simulink model "Simulation_model_islanded"  (R2021a)
settings: Solver=ode23t  StartTime=0.0  StopTime=6  FixedStep=T  RelTol=1e-3
values from neighbouring files (symbols this model uses):
  C_dc = Cb*c_dc_pu    [parameters.m]
  C_f = Cb*c_f_pu    [parameters.m]
  f_SM = fb    (= 50)    [parameters.m]
  fb = 50    [parameters.m]
  ff_SM = 0.01322    [parameters.m]
  Ib = 2/3*Sb/Vb    [parameters.m]
  Ib_dc = Sb/Vb_dc    [parameters.m]
  ic_SM = 0.8    [parameters.m]
  K_ad = 1.5    [parameters.m]
  K_ffv = 0    [parameters.m]
  K_ic = K_pc/T_1    [parameters.m]
  K_idc = K_pdc/T_idc    (= 250)    [parameters.m]
  K_iPLL = a^2*T_fPLL    (= 0.09)    [parameters.m]
  K_iv = K_pv/T_iv    (= 92.0050761421)    [parameters.m]
  K_iv_SM = K_pv_SM/T_iv_SM    (= 70)    [parameters.m]
  K_omega = 20    [parameters.m]
  K_omega_SM = 40    [parameters.m]
  K_pc = l_f_pu/(4*pi*fb*T_sum)    (= 1.27323954474)    [parameters.m]
  K_pdc = 25    [parameters.m]
  K_pPLL = 1/(a*2*pi*T_fPLL)    (= 5.30516476973)    [parameters.m]
  K_pv = 0.29    [parameters.m]
  K_pv_SM = 35    [parameters.m]
  K_vco = 2*pi    (= 6.28318530718)    [parameters.m]
  Kd = 40    [parameters.m]
  Kq = 0.1    [parameters.m]
  Kq_SM = 0.1    [parameters.m]
  L_f = Lb*l_f_pu    [parameters.m]
  l_f_pu = 0.08    [parameters.m]
  lf1f = 0    [parameters.m]
  lfd_SM = 0.531    [parameters.m]
  llkd = 2.655    [parameters.m]
  llkq1 = 0.2408    [parameters.m]
  lls_SM = 0.08    [parameters.m]
  lmd_SM = 2.81    [parameters.m]
  lmq_SM = 1.64    [parameters.m]
  omega_ad = 50    [parameters.m]
  omega_b = 2*pi*fb    (= 314.159265359)    [parameters.m]
  omega_d = 5    [parameters.m]
  omega_qf = 200    [parameters.m]
  omega_qf_SM = 200    [parameters.m]
  omega_vf = 200    [parameters.m]
  p_h = 0.1    [parameters.m]
  pp_SM = 2    [parameters.m]
  R_lf = Rb*r_lf_pu    [parameters.m]
  rfd_SM = 0.004319    [parameters.m]
  rkd = 0.2343    [parameters.m]
  rkq1 = 0.03365    [parameters.m]
  rs_SM = 0.01524    [parameters.m]
  S_SM = Sb    (= 1000000)    [parameters.m]
  Sb = 1e6    (= 1000000)    [parameters.m]
  T = 1e-4    (= 0.0001)    [parameters.m]
  T_fPLL = 10e-3    (= 0.01)    [parameters.m]
  T_gt_SM = 0.5    [parameters.m]
  Ta = 4    [parameters.m]
  v_dc_ref = 1    [parameters.m]
  V_SM = V    (= 690)    [parameters.m]
  Vb = V*sqrt(2)/sqrt(3)    [parameters.m]
  Vb_dc = Vb*2    [parameters.m]
undefined symbols (not defined in the file or in its folder): D11, Delta
libraries: simulink_extras x18, spsDiodeLib x12, spsThreePhaseVIMeasurementLib x9, spsThreePhaseSeriesRLCBranchLib x7, spsPower3phInstantaneousLib x5, spsVoltageMeasurementLib x3, spsControlledCurrentSourceLib x2, spsThreePhaseParallelRLCLoadLib x2, spsThreePhaseBreakerLib x2, spsUniversalBridgeLib x2, spsDCVoltageSourceLib x1, spsGroundLib x1
(part 1 of 2)
settings Model: Creator=HLunn  LastModifiedBy=HLunn

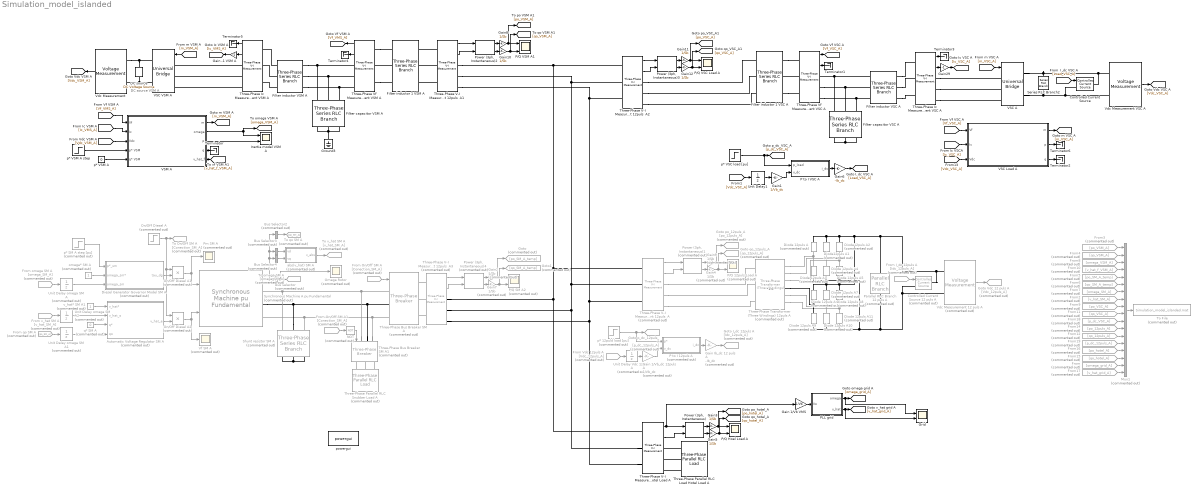
== system Simulation_model_islanded ==
  note: *1.6
  note: DC source
      | VSM A
  Automatic Voltage Regulator SM A : Subsystem  Commented=on
  Bus Selector : BusSelector  Commented=on  OutputSignals="Mechanical.Rotor speed  wm (pu)"  OutputAsBus=on
  Bus Selector2 : BusSelector  Commented=on  OutputSignals="Output reactive power  Qeo (pu)"  OutputAsBus=on
  Bus Selector3 : BusSelector  Commented=on  OutputSignals="dq0 components.Stator voltage  vd (pu)"  OutputAsBus=on
  Bus Selector4 : BusSelector  Commented=on  OutputSignals="dq0 components.Stator voltage  vq (pu)"  OutputAsBus=on
  Controlled Current Source : spsControlledCurrentSourceLib/Controlled Current Source  Initialize=on  Source_Type=DC  Amplitude=0  Phase=0  Frequency=0  Measurements=None
  Controlled Current Source 12 puls A : spsControlledCurrentSourceLib/Controlled Current Source  Commented=on  Initialize=on  Source_Type=DC  Amplitude=0  Phase=0  Frequency=0  Measurements=None
  DC source : spsDCVoltageSourceLib/DC Voltage Source  Amplitude=Vb_dc  Measurements=None
  Diesel Generator Governor Model SM A : Subsystem  Commented=on
  Diode 12puls A{,3..11} (10 alike) : spsDiodeLib/Diode  Commented=on  Ron=0.001  Lon=0  Vf=0.8  IC=0  UseSnubber=0  Rs=500  Cs=250e-9  Measurements=off
  Diode12puls A1 : spsDiodeLib/Diode  Commented=on  Ron=0.001  Lon=0  Vf=0.8  IC=0  UseSnubber=0  Rs=500  Cs=250e-9  Measurements=off
  Diode12puls A2 : spsDiodeLib/Diode  Commented=on  Ron=0.001  Lon=0  Vf=0.8  IC=0  UseSnubber=0  Rs=500  Cs=250e-9  Measurements=off
  Filter capacitor VSC A : spsThreePhaseSeriesRLCBranchLib/Three-Phase Series RLC Branch  LConnTagsString=A|B|C  RConnTagsString=A|B|C  BranchType=RC  Resistance=R_lf  Inductance=L_f  Capacitance=C_f  Measurements=None
  Filter capacitor VSM A : spsThreePhaseSeriesRLCBranchLib/Three-Phase Series RLC Branch  LConnTagsString=A|B|C  RConnTagsString=A|B|C  BranchType=RC  Resistance=R_lf  Inductance=L_f  Capacitance=C_f  Measurements=None
  Filter inductor VSC A : spsThreePhaseSeriesRLCBranchLib/Three-Phase Series RLC Branch  LConnTagsString=A|B|C  RConnTagsString=A|B|C  BranchType=RL  Resistance=R_lf  Inductance=L_f  Capacitance=1e-6  Measurements=None
  Filter inductor VSM A : spsThreePhaseSeriesRLCBranchLib/Three-Phase Series RLC Branch  LConnTagsString=A|B|C  RConnTagsString=A|B|C  BranchType=RL  Resistance=R_lf  Inductance=L_f  Capacitance=1e-6  Measurements=None
  Filter inductor 1 VSC A : spsThreePhaseSeriesRLCBranchLib/Three-Phase Series RLC Branch  LConnTagsString=A|B|C  RConnTagsString=A|B|C  BranchType=RL  Resistance=R_lf  Inductance=L_f  Capacitance=1e-6  Measurements=None
  Filter inductor 1 VSM A : spsThreePhaseSeriesRLCBranchLib/Three-Phase Series RLC Branch  LConnTagsString=A|B|C  RConnTagsString=A|B|C  BranchType=RL  Resistance=R_lf  Inductance=L_f  Capacitance=1e-6  Measurements=None
  From : From  Commented=on  GotoTag=omega_grid_A
  From I_dc 12puls A : From  Commented=on  GotoTag=Idc_12puls_A
  From On/Off SM A : From  Commented=on  GotoTag=Conection_SM_A
  From On/Off SM A1 : From  Commented=on  GotoTag=Conection_SM_A
  From Vdc 12puls A : From  Commented=on  GotoTag=Vdc_12puls_A
  From omega SM A : From  Commented=on  GotoTag=omega_SM_A
  From qo SM A : From  Commented=on  GotoTag=qo_SM_A
  From v_hat SM A : From  Commented=on  GotoTag=v_hat_SM_A
  From10 : From  Commented=on  GotoTag=v_hat_f_VSM_A
  From11 : From  Commented=on  GotoTag=qo_VSC_A
  From12 : From  Commented=on  GotoTag=qo_12puls_A
  From14 : From  Commented=on  GotoTag=po_12puls_A
  From15 : From  Commented=on  GotoTag=qo_hotel_A
  From16 : From  Commented=on  GotoTag=po_hotel_A
  From17 : From  Commented=on  GotoTag=v_hat_grid_A
  From18 : From  Commented=on  GotoTag=p_dc_VSC_A
  From19 : From  Commented=on  GotoTag=p_dc_12puls_A
  From2 : From  Commented=on  GotoTag=v_hat_SM_A
  From3 : From  Commented=on  GotoTag=po_VSM_A
  From4 : From  Commented=on  GotoTag=qo_VSM_A
  From5 : From  Commented=on  GotoTag=po_SM_A_temp
  From6 : From  Commented=on  GotoTag=qo_SM_A_temp
  From7 : From  Commented=on  GotoTag=omega_SM_A
  From8 : From  Commented=on  GotoTag=omega_VSM_A
  From9 : From  Commented=on  GotoTag=po_VSC_A
  Gain -1 VSM A : Gain  Gain=-1
  Gain 1/Vb VMS : Gain  Gain=1/Vb
  Gain 1/Vb_dc 12puls A : Gain  Commented=on  Gain=1/Vb_dc
  Gain Ib_dc 12 puls A : Gain  Commented=on  Gain=-Ib_dc
  Gain1 : Gain  Gain=1/Vb_dc
  Gain{3,5,8,10..12} (6 alike) : Gain  Gain=1/Sb
  Gain{2,4,7,9} (4 alike) : Gain  Commented=on  Gain=1/Sb
  Gain29 : Gain  Gain=-1
  Gain6 : Gain  Gain=-Ib_dc
  Goto : Goto  Commented=on  GotoTag=po_SM_A_temp
  Goto I_dc 12puls A : Goto  Commented=on  GotoTag=Idc_12puls_A
  Goto Vdc 12 puls A : Goto  Commented=on  GotoTag=Vdc_12puls_A
  Goto p_dc_12puls_A : Goto  Commented=on  GotoTag=p_dc_12puls_A
  Goto po_12puls_A : Goto  Commented=on  GotoTag=po_12puls_A
  Goto qo_12puls_A : Goto  Commented=on  GotoTag=qo_12puls_A
  Goto1 : Goto  Commented=on  GotoTag=qo_SM_A_temp
  Grid : Scope  NumInputPorts=2
  Ground3 : spsGroundLib/Ground  LConnTagsString=a
  Inertia model VSM A : Scope  NumInputPorts=2
  Mux1 : Mux  Commented=on  Inputs=18
  NOT : Logic  Commented=on  Operator=NOT  IconShape=distinctive  AllPortsSameDT=off  OutDataTypeStr=boolean
  Omega Rotor : Scope  Commented=on
  On/Off Diesel A : Step  Commented=on  Time=4.002  Before=1  After=0  SampleTime=0
  On/Off Diesel A1 : Product  Commented=on  Inputs=**
  On/Off Diesel A2 : Product  Commented=on  Inputs=**
  P to I VSC A : Subsystem
  P to I 12puls A : Subsystem  Commented=on
  P/Q 12puls Load A : Scope  Commented=on  NumInputPorts=2
  P/Q Hoel Load A : Scope  NumInputPorts=2
  P/Q SM A2 : Scope  Commented=on  NumInputPorts=2
  P/Q VSC Load A : Scope  NumInputPorts=2
  P/Q VSM A1 : Scope  NumInputPorts=2
  PLL grid : Subsystem
  Parallel RLC Branch 12 puls A : spsParallelRLCBranchLib/Parallel RLC Branch  Commented=on  LConnTagsString=a  RConnTagsString=__new0  BranchType=C  Resistance=1e3  Inductance=1e-3  SetiL0=off  InitialCurrent=0  Capacitance=C_dc  Setx0=on  InitialVoltage=Vb_dc  Measurements=None
  Pm SM A : Scope  Commented=on
  "Power (3ph, Instantaneous)" : spsPower3phInstantaneousLib/Power (3ph, Instantaneous)
  "Power (3ph, Instantaneous)1" : spsPower3phInstantaneousLib/Power (3ph, Instantaneous)  Commented=on
  "Power (3ph, Instantaneous)2" : spsPower3phInstantaneousLib/Power (3ph, Instantaneous)
  "Power (3ph, Instantaneous)3" : spsPower3phInstantaneousLib/Power (3ph, Instantaneous)
  "Power (3ph, Instantaneous)4" : spsPower3phInstantaneousLib/Power (3ph, Instantaneous)  Commented=on
  Series RLC Branch2 : spsSeriesRLCBranchLib/Series RLC Branch  LConnTagsString=__new0  RConnTagsString=__new0  BranchType=C  Resistance=0  Inductance=0  SetiL0=off  InitialCurrent=0  Capacitance=C_dc  Setx0=on  InitialVoltage=Vb_dc  Measurements=None
  Shunt resistor SM A : spsThreePhaseSeriesRLCBranchLib/Three-Phase Series RLC Branch  Commented=on  LConnTagsString=A|B|C  RConnTagsString=A|B|C  BranchType=R  Resistance=1e6  Inductance=L_f  Capacitance=C_f  Measurements=None
  Synchronous Machine A pu Fundamental : spsSynchronousMachinepuFundamentalLib/Synchronous Machine pu Fundamental  Commented=on  PresetModel=No  MechanicalLoad=Mechanical power Pm  ShowDetailedParameters=on  RotorType=Salient-pole  Units=per unit fundamental parameters  MeasurementBus=off  NominalParameters=[S_SM V_SM f_SM]  Stator=[rs_SM lls_SM lmd_SM lmq_SM lf1f]  Field=[rfd_SM lfd_SM]  Dampers2=[0.0652, 0.5134, 0.0287, 0.2553, 7.765e-3, 0.9167 ]  Dampers1=[rkd llkd rkq1 llkq1]  Mechanical=[ic_SM ff_SM pp_SM]  PolePairs=20  InitialConditions="[ 0  0  0  0  0  0  0  0  1 ]"  SetSaturation=off  Saturation=[0.6404,0.7127,0.8441,0.9214,0.9956,1.082,1.19,1.316,1.457;0.7,0.7698,0.8872,0.9466,0.9969,1.046,1.1,1.151,1.201]  LoadFlowParameters=[1,0,0,0,0]  TsPowergui=0  TsBlock=-1  IterativeModel=Trapezoidal non iterative  IterativeDiscreteModel=Trapezoidal non iterative  BusType=PV  Pref=0  Qref=0  Qmin=-inf  Qmax=inf  PLF=0  QLF=0
      settings: SourceProductBaseCode=PS
  Terminator{,1..6} (7 alike) : Terminator
  Three-Phase Ic Measurement VSC A : spsThreePhaseVIMeasurementLib/Three-Phase V-I Measurement  VoltageMeasurement=phase-to-ground  SetLabelV=off  LabelV=V_cv  Vpu=off  VpuLL=off  CurrentMeasurement=yes  SetLabelI=off  LabelI=I_cv  Ipu=off  Pbase=Sb  Vbase=V  OutputType=Complex  PhasorSimulation=off  PSBequivalent=0
  Three-Phase Ic Measurement VSM A : spsThreePhaseVIMeasurementLib/Three-Phase V-I Measurement  VoltageMeasurement=phase-to-ground  SetLabelV=off  LabelV=V_cv  Vpu=off  VpuLL=off  CurrentMeasurement=yes  SetLabelI=off  LabelI=I_cv  Ipu=off  Pbase=Sb  Vbase=V  OutputType=Complex  PhasorSimulation=off  PSBequivalent=0
  Three-Phase Parallel RLC Snubber Load A : spsThreePhaseParallelRLCLoadLib/Three-Phase Parallel RLC Load  Commented=on  LConnTagsString=A|B|C  Configuration=Y (floating)  NominalVoltage=690  Vabc=[1e3 1e3 1e3]  Vabcp=[1e3 1e3 1e3]  NominalFrequency=50  UnbalancedPower=off  ActivePower=Sb*0.5  InductivePower=0  CapacitivePower=0  Pabc=[10e3 9e3 11e3]  QLabc=[100 90 110]  QCabc=[100 90 110]  Pabcp=[10e3 9e3 11e3]  QLabcp=[100 90 110]  QCabcp=[100 90 110]  Measurements=None  LoadType=constant Z
  Three-Phase Parallel RLC Load Hotel Load A : spsThreePhaseParallelRLCLoadLib/Three-Phase Parallel RLC Load  LConnTagsString=A|B|C  Configuration=Y (floating)  NominalVoltage=690  Vabc=[1e3 1e3 1e3]  Vabcp=[1e3 1e3 1e3]  NominalFrequency=fb  UnbalancedPower=off  ActivePower=Sb*p_h  InductivePower=0  CapacitivePower=0  Pabc=[10e3 9e3 11e3]  QLabc=[100 90 110]  QCabc=[100 90 110]  Pabcp=[10e3 9e3 11e3]  QLabcp=[100 90 110]  QCabcp=[100 90 110]  Measurements=None  LoadType=constant Z
  Three-Phase Transformer (Three Windings) 12puls A : spsThreePhaseTransformerThreeWindingsLib/Three-Phase Transformer (Three Windings)  Commented=on  Winding1Connection=Y  Winding2Connection=Y  Winding3Connection=Delta (D11)  CoreType=Three single-phase transformers  SetSaturation=off  Hysteresis=off  DataFile='hysteresis'  SetInitialFlux=off  Measurements=None  UNITS=pu  NominalPower=[Sb , fb]  Winding1=[690 0.005 0.04]  Winding2=[690 0.005 0.03]  Winding3=[690 0.005 0.03]  Rm=100  Lm=100  L0=0.5  Saturation=[0 0;2.2531e-06 1278.3;0.00093879 1619.1]  InitialFluxes=[0.8 -0.8 0.7]  BreakLoop=off  DiscreteSolver=Trapezoidal iterative  DataType=off  TransfoNumber=1
      settings: SourceProductBaseCode=PS
  Three-Phase V-I Measurement 12puls  A : spsThreePhaseVIMeasurementLib/Three-Phase V-I Measurement  Commented=on  VoltageMeasurement=phase-to-ground  SetLabelV=off  LabelV=Vabc  Vpu=off  VpuLL=off  CurrentMeasurement=yes  SetLabelI=off  LabelI=Iabc  Ipu=off  Pbase=100e6  Vbase=500e3  OutputType=Complex  PhasorSimulation=off  PSBequivalent=0
  Three-Phase V-I Measurement 12puls  A1 : spsThreePhaseVIMeasurementLib/Three-Phase V-I Measurement  VoltageMeasurement=phase-to-ground  SetLabelV=off  LabelV=Vabc  Vpu=off  VpuLL=off  CurrentMeasurement=yes  SetLabelI=off  LabelI=Iabc  Ipu=off  Pbase=100e6  Vbase=500e3  OutputType=Complex  PhasorSimulation=off  PSBequivalent=0
  Three-Phase V-I Measurement 12puls  A2 : spsThreePhaseVIMeasurementLib/Three-Phase V-I Measurement  VoltageMeasurement=phase-to-ground  SetLabelV=off  LabelV=Vabc  Vpu=off  VpuLL=off  CurrentMeasurement=yes  SetLabelI=off  LabelI=Iabc  Ipu=off  Pbase=100e6  Vbase=500e3  OutputType=Complex  PhasorSimulation=off  PSBequivalent=0
  Three-Phase V-I Measurement 12puls  A3 : spsThreePhaseVIMeasurementLib/Three-Phase V-I Measurement  Commented=on  VoltageMeasurement=phase-to-ground  SetLabelV=off  LabelV=Vabc  Vpu=off  VpuLL=off  CurrentMeasurement=yes  SetLabelI=off  LabelI=Iabc  Ipu=off  Pbase=100e6  Vbase=500e3  OutputType=Complex  PhasorSimulation=off  PSBequivalent=0
  Three-Phase V-I Measurement Hotel Load A : spsThreePhaseVIMeasurementLib/Three-Phase V-I Measurement  VoltageMeasurement=phase-to-ground  SetLabelV=off  LabelV=Vabc  Vpu=off  VpuLL=off  CurrentMeasurement=yes  SetLabelI=off  LabelI=Iabc  Ipu=off  Pbase=100e6  Vbase=500e3  OutputType=Complex  PhasorSimulation=off  PSBequivalent=0
  Three-Phase Vf Measurement VSC A : spsThreePhaseVIMeasurementLib/Three-Phase V-I Measurement  VoltageMeasurement=phase-to-ground  SetLabelV=off  LabelV=Vabc  Vpu=off  VpuLL=off  CurrentMeasurement=yes  SetLabelI=off  LabelI=Iabc  Ipu=off  Pbase=100e6  Vbase=500e3  OutputType=Complex  PhasorSimulation=off  PSBequivalent=0
  Three-Phase Vf Measurement VSM A : spsThreePhaseVIMeasurementLib/Three-Phase V-I Measurement  VoltageMeasurement=phase-to-ground  SetLabelV=off  LabelV=Vabc  Vpu=off  VpuLL=off  CurrentMeasurement=yes  SetLabelI=off  LabelI=Iabc  Ipu=off  Pbase=100e6  Vbase=500e3  OutputType=Complex  PhasorSimulation=off  PSBequivalent=0
  Three-Phase Bus Breaker SM A : spsThreePhaseBreakerLib/Three-Phase Breaker  Commented=on  InitialState=closed  SwitchA=on  SwitchB=on  SwitchC=on  SwitchTimes=[1]  External=on  BreakerResistance=0.01  SnubberResistance=1e6  SnubberCapacitance=inf  Measurements=None
  Three-Phase Bus Breaker SM A1 : spsThreePhaseBreakerLib/Three-Phase Breaker  Commented=on  InitialState=open  SwitchA=on  SwitchB=on  SwitchC=on  SwitchTimes=[1]  External=on  BreakerResistance=0.01  SnubberResistance=1e6  SnubberCapacitance=inf  Measurements=None
  To File : ToFile  Commented=on  Filename=Simulation_model_islanded.mat  MatrixName=Simulation_model_islanded
  To On/Off SM A : Goto  Commented=on  GotoTag=Conection_SM_A
  To omega SM A : Goto  Commented=on  GotoTag=omega_SM_A
  To qo SM A : Goto  Commented=on  GotoTag=qo_SM_A
  To v_hat SM A : Goto  Commented=on  GotoTag=v_hat_SM_A
  Unit Delay Vdc 12puls A : UnitDelay  Commented=on  InitialCondition=Vb_dc  SampleTime=-1  HasFrameUpgradeWarning=on
  Unit Delay omega SM A : UnitDelay  Commented=on  SampleTime=-1  HasFrameUpgradeWarning=on
  Unit Delay omega SM A1 : UnitDelay  Commented=on  SampleTime=-1  HasFrameUpgradeWarning=on
  Unit Delay omega SM A2 : UnitDelay  Commented=on  SampleTime=-1  HasFrameUpgradeWarning=on
  Unit Delay1 : UnitDelay  InitialCondition=Vb_dc  SampleTime=-1  HasFrameUpgradeWarning=on
  VSC A : spsUniversalBridgeLib/Universal Bridge  Arms=3  SnubberResistance=1e5  SnubberCapacitance=inf  Device=Average-model based VSC  Ron=1e-3  Lon=0  ForwardVoltages="[  0  0  ]"  ForwardVoltage=0  GTOparameters=[ 10e-6 , 20e-6 ]  IGBTparameters=[ 1e-6 , 2e-6 ]  Measurements=None  Measurements_2=None  converterType=Rectifier
  VSC Load A : Subsystem
  VSC VSM A : spsUniversalBridgeLib/Universal Bridge  Arms=3  SnubberResistance=1e5  SnubberCapacitance=inf  Device=Average-model based VSC  Ron=1e-3  Lon=0  ForwardVoltages="[  0  0  ]"  ForwardVoltage=0  GTOparameters=[ 10e-6 , 20e-6 ]  IGBTparameters=[ 1e-6 , 2e-6 ]  Measurements=None  Measurements_2=None  converterType=Rectifier
  VSM A : Subsystem
  Vdc Measurement : spsVoltageMeasurementLib/Voltage Measurement  PhasorSimulation=off  OutputType=Complex  PSBequivalent=0
  Vdc Measurement 12 puls A : spsVoltageMeasurementLib/Voltage Measurement  Commented=on  PhasorSimulation=off  OutputType=Complex  PSBequivalent=0
  Vdc Measurement VSC A : spsVoltageMeasurementLib/Voltage Measurement  PhasorSimulation=off  OutputType=Complex  PSBequivalent=0
  Vf SM A : Scope  Commented=on
  abs(v_hat) SM A : MATLAB Function  Commented=on  TreatAsAtomicUnit=on
  omega* SM A : Constant  Commented=on
  p* 12puld load [pu] : Step  Commented=on  Time=2  After=0.3  SampleTime=0
  p* SM A step [pu] : Step  Commented=on  Time=2  Before=0.4  After=0  SampleTime=0
  p* VSC load [pu] : Step  Time=2  After=0.3  SampleTime=0
  p* VSM A : Constant  Value=0
  p* VSM A step : Step  Time=2  Before=0.1  After=0.4  SampleTime=0
  powergui : spspowerguiLib/powergui  Priority=1  SimulationMode=Discrete  SampleTime=T  frequency=60  Iterations=50  frequencyindice=0  Pbase=100e6  ErrMax=1e-4  UnitsV=kV  UnitsW=MW  buscounter=0  FunctionMessages=off  echomessages=off  EnableUseOfTLC=off  CurrentSourceSwitches=off  DisableSnubberDevices=off  DisableRonSwitches=off  DisableVfSwitches=off  DisplayEquations=off  AutomaticDiscreteSolvers=off  SolverType=Tustin/Backward Euler (TBE)  Interpol=off  ExternalGateDelay=off  methode=off  Ts=100  x0status=blocks  SPID=on  SwTol=0  HookPort=off  NonlinearTolerance=1e-4  nMaxIteration=100  ContinueOnMaxIteration=off  RestoreLinks=warning  ResistiveCurrentMeasurement=off  Frange=[0:2:500]  Ylog=off  Xlog=on  ShowGrid=off  save=off  variable=ZData  structure=0  ZoomFFT=off  StartTime=0.0  cycles=1  DisplayStyle=1  fundamental=60  FreqAxis=off  MaxFrequency=1000  frequencyindicesteady=1  RmsSteady=1  display=off
  q* SM A : Constant  Commented=on  Value=0
  v_hat* SM A1 : Constant  Commented=on
  wires:
  [m_VSM_A] -> VSC VSM A/1
  Three-Phase Ic Measurement VSM A/1 -> Terminator5/1
  Three-Phase Vf Measurement VSM A/2 -> Terminator4/1
  Three-Phase Ic Measurement VSM A/2 -> Gain -1 VSM A/1
  Three-Phase Vf Measurement VSM A/1 -> [Vf_VMS_A]
  VSM A/1(m) -> [m_VSM_A]
  [Vdc_VSC_A] -> Unit Delay1/1
  Vdc Measurement/1 -> [Vdc_VSM_A]
  [Ic_VSC_A] -> VSC Load A/2(Ic)
  [Vf_VSC_A] -> VSC Load A/1(Vf)
  Gain1/1 -> P to I VSC A/2(v_dc)
  [Vdc_VSC_A] -> VSC Load A/3(Vdc)
  Gain6/1 -> [Load_VSC_A]
  Unit Delay Vdc 12puls A/1 -> Gain 1/Vb_dc 12puls A/1
  [m_VSC_A] -> VSC A/1
  [Load_VSC_A] -> Controlled Current Source/1
  Gain Ib_dc 12 puls A/1 -> Goto I_dc 12puls A/1
  From Vdc 12puls A/1 -> Unit Delay Vdc 12puls A/1
  Three-Phase Ic Measurement VSC A/2 -> Gain29/1
  Three-Phase Vf Measurement VSC A/1 -> [Vf_VSC_A]
  Vdc Measurement VSC A/1 -> [Vdc_VSC_A]
  From I_dc 12puls A/1 -> Controlled Current Source 12 puls A/1
  Unit Delay1/1 -> Gain1/1
  Three-Phase Vf Measurement VSC A/2 -> Terminator1/1
  Gain 1/Vb_dc 12puls A/1 -> P to I 12puls A/2(v_dc)
  P to I 12puls A/1(i_dc) -> Gain Ib_dc 12 puls A/1
  Vdc Measurement 12 puls A/1 -> Goto Vdc 12 puls A/1
  Three-Phase Ic Measurement VSC A/1 -> Terminator3/1
  P to I VSC A/1(i_dc) -> Gain6/1
  VSM A/2(omega) -> Inertia model VSM A/1, [omega_VSM_A]
  VSM A/3(p) -> Inertia model VSM A/2
  [Ic_VMS_A] -> VSM A/2(Ic)
  [Vf_VMS_A] -> VSM A/1(Vf)
  [Vdc_VSM_A] -> VSM A/3(Vdc)
  VSC Load A/1(m) -> [m_VSC_A]
  VSC Load A/2(p) -> Terminator6/1
  VSC Load A/3(q) -> Terminator2/1
  NOT/1 -> Three-Phase Bus Breaker SM A1/1
  omega* SM A/1 -> Diesel Generator Governor Model SM A/2(omega_sm*)
  Unit Delay omega SM A1/1 -> Automatic Voltage Regulator SM A/4(qo)
  Diesel Generator Governor Model SM A/1(tau_dg) -> On/Off Diesel A1/2
  Bus Selector4/1 -> abs(v_hat) SM A/2(vq)
  From omega SM A/1 -> Unit Delay omega SM A/1
  On/Off Diesel A1/1 -> Pm SM A/1, Synchronous Machine A pu Fundamental/1
  From v_hat SM A/1 -> Unit Delay omega SM A2/1
  q* SM A/1 -> Automatic Voltage Regulator SM A/3(q*)
  Unit Delay omega SM A/1 -> Diesel Generator Governor Model SM A/3(omega_sm)
  From qo SM A/1 -> Unit Delay omega SM A1/1
  Synchronous Machine A pu Fundamental/1 -> Bus Selector/1, Bus Selector2/1, Bus Selector3/1, Bus Selector4/1
  From On/Off SM A/1 -> Three-Phase Bus Breaker SM A/1
  Bus Selector/1 -> Omega Rotor/1, To omega SM A/1
  From On/Off SM A1/1 -> NOT/1
  abs(v_hat) SM A/1(v_abs) -> To v_hat SM A/1
  Bus Selector3/1 -> abs(v_hat) SM A/1(vd)
  Unit Delay omega SM A2/1 -> Automatic Voltage Regulator SM A/2(v_hat_o)
  v_hat* SM A1/1 -> Automatic Voltage Regulator SM A/1(v_hat*)
  Automatic Voltage Regulator SM A/1(v_hat_e) -> On/Off Diesel A2/2
  On/Off Diesel A2/1 -> Vf SM A/1, Synchronous Machine A pu Fundamental/2
  On/Off Diesel A/1 -> On/Off Diesel A2/1, On/Off Diesel A1/1, To On/Off SM A/1
  Gain29/1 -> [Ic_VSC_A]
  Gain -1 VSM A/1 -> [Ic_VMS_A]
  Bus Selector2/1 -> To qo SM A/1
  Three-Phase V-I Measurement Hotel Load A/2 -> "Power (3ph, Instantaneous)"/2
  "Power (3ph, Instantaneous)"/1 -> Gain3/1
  "Power (3ph, Instantaneous)"/2 -> Gain5/1
  Gain3/1 -> P/Q Hoel Load A/1, [po_hotel_A]
  Gain5/1 -> P/Q Hoel Load A/2, [qo_hotel_A]
  Three-Phase V-I Measurement 12puls  A/2 -> "Power (3ph, Instantaneous)1"/2
  "Power (3ph, Instantaneous)1"/2 -> Gain9/1
  Three-Phase V-I Measurement 12puls  A/1 -> "Power (3ph, Instantaneous)1"/1
  "Power (3ph, Instantaneous)1"/1 -> Gain4/1
  Gain4/1 -> P/Q 12puls Load A/1, Goto po_12puls_A/1
  Gain9/1 -> P/Q 12puls Load A/2, Goto qo_12puls_A/1
  Mux1/1 -> To File/1
  VSM A/5(v_hat_f) -> [v_hat_f_VSM_A]
  From3/1 -> Mux1/1
  From4/1 -> Mux1/2
  From8/1 -> Mux1/3
  From10/1 -> Mux1/4
  From5/1 -> Mux1/5
  From6/1 -> Mux1/6
  From7/1 -> Mux1/7
  From2/1 -> Mux1/8
  From9/1 -> Mux1/9
  From11/1 -> Mux1/10
  Gain 1/Vb VMS/1 -> PLL grid/1(Vo)
  Three-Phase V-I Measurement Hotel Load A/1 -> Gain 1/Vb VMS/1, "Power (3ph, Instantaneous)"/1
  PLL grid/1(omega) -> Grid/1, [omega_grid_A]
  PLL grid/2(v_hat) -> Grid/2, [v_hat_grid_A]
  From14/1 -> Mux1/12
  From16/1 -> Mux1/15
  From15/1 -> Mux1/16
  From17/1 -> Mux1/18
  From/1 -> Mux1/17
  From18/1 -> Mux1/11
  From19/1 -> Mux1/14
  From12/1 -> Mux1/13
  p* 12puld load [pu]/1 -> P to I 12puls A/1(p*), Goto p_dc_12puls_A/1
  Gain10/1 -> [qo_VSM_A], P/Q VSM A1/2
  Gain8/1 -> [po_VSM_A], P/Q VSM A1/1
  "Power (3ph, Instantaneous)2"/1 -> Gain8/1
  Three-Phase V-I Measurement 12puls  A1/1 -> "Power (3ph, Instantaneous)2"/1
  "Power (3ph, Instantaneous)2"/2 -> Gain10/1
  Three-Phase V-I Measurement 12puls  A1/2 -> "Power (3ph, Instantaneous)2"/2
  Gain12/1 -> [qo_VSC_A], P/Q VSC Load A/2
  Gain11/1 -> [po_VSC_A], P/Q VSC Load A/1
  "Power (3ph, Instantaneous)3"/1 -> Gain11/1
  Three-Phase V-I Measurement 12puls  A2/1 -> "Power (3ph, Instantaneous)3"/1
  "Power (3ph, Instantaneous)3"/2 -> Gain12/1
  Three-Phase V-I Measurement 12puls  A2/2 -> "Power (3ph, Instantaneous)3"/2
  Gain7/1 -> Goto/1, P/Q SM A2/1
  "Power (3ph, Instantaneous)4"/2 -> Gain2/1
  Three-Phase V-I Measurement 12puls  A3/1 -> "Power (3ph, Instantaneous)4"/1
  Gain2/1 -> Goto1/1, P/Q SM A2/2
  Three-Phase V-I Measurement 12puls  A3/2 -> "Power (3ph, Instantaneous)4"/2
  "Power (3ph, Instantaneous)4"/1 -> Gain7/1
  p* VSM A/1 -> VSM A/5(q* VSM)
  p* VSM A step/1 -> VSM A/4(p* VSM)
  p* VSC load [pu]/1 -> P to I VSC A/1(p_load), [p_dc_VSC_A]
  p* SM A step [pu]/1 -> Diesel Generator Governor Model SM A/1(p*_sm)
  VSM A/4(q) -> Terminator/1
  connections:
  DC source/LConn1 -- Vdc Measurement/LConn2 -- VSC VSM A/RConn2
  Three-Phase Transformer (Three Windings) 12puls A/RConn1 -- Diode 12puls A3/RConn1 -- Diode 12puls A/LConn1
  Diode 12puls A4/LConn1 -- Diode 12puls A3/LConn1 -- Parallel RLC Branch 12 puls A/RConn1 -- Controlled Current Source 12 puls A/LConn1 -- Vdc Measurement 12 puls A/LConn2 -- Diode 12puls A11/LConn1 -- Diode 12puls A9/LConn1 -- Diode 12puls A10/LConn1 -- Diode 12puls A5/LConn1
  Filter inductor VSC A/LConn3 -- Three-Phase Vf Measurement VSC A/RConn3 -- Filter capacitor VSC A/LConn3
  Vdc Measurement VSC A/LConn2 -- Controlled Current Source/LConn1 -- Series RLC Branch2/RConn1 -- VSC A/RConn2
  Filter inductor VSM A/LConn2 -- Three-Phase Vf Measurement VSM A/RConn2 -- Filter capacitor VSM A/LConn2
  Filter inductor VSC A/LConn2 -- Three-Phase Vf Measurement VSC A/RConn2 -- Filter capacitor VSC A/LConn2
  Filter capacitor VSM A/RConn3 -- Ground3/LConn1 -- Filter capacitor VSM A/RConn1 -- Filter capacitor VSM A/RConn2
  Diode 12puls A8/LConn1 -- Three-Phase Transformer (Three Windings) 12puls A/RConn6 -- Diode 12puls A11/RConn1
  Three-Phase Transformer (Three Windings) 12puls A/RConn2 -- Diode 12puls A4/RConn1 -- Diode12puls A1/LConn1
  Three-Phase Transformer (Three Windings) 12puls A/RConn5 -- Diode 12puls A7/LConn1 -- Diode 12puls A10/RConn1
  Filter inductor VSM A/LConn1 -- Three-Phase Vf Measurement VSM A/RConn1 -- Filter capacitor VSM A/LConn1
  DC source/RConn1 -- VSC VSM A/RConn1 -- Vdc Measurement/LConn1
  Series RLC Branch2/LConn1 -- Controlled Current Source/RConn1 -- Vdc Measurement VSC A/LConn1 -- VSC A/RConn1
  Three-Phase Vf Measurement VSC A/RConn1 -- Filter inductor VSC A/LConn1 -- Filter capacitor VSC A/LConn1
  Diode 12puls A5/RConn1 -- Three-Phase Transformer (Three Windings) 12puls A/RConn3 -- Diode12puls A2/LConn1
  Diode 12puls A6/RConn1 -- Diode 12puls A7/RConn1 -- Parallel RLC Branch 12 puls A/LConn1 -- Controlled Current Source 12 puls A/RConn1 -- Vdc Measurement 12 puls A/LConn1 -- Diode12puls A2/RConn1 -- Diode 12puls A/RConn1 -- Diode12puls A1/RConn1 -- Diode 12puls A8/RConn1
  Filter inductor VSM A/LConn3 -- Three-Phase Vf Measurement VSM A/RConn3 -- Filter capacitor VSM A/LConn3
  Diode 12puls A9/RConn1 -- Diode 12puls A6/LConn1 -- Three-Phase Transformer (Three Windings) 12puls A/RConn4
  Filter capacitor VSC A/RConn3 -- Filter capacitor VSC A/RConn2 -- Filter capacitor VSC A/RConn1
  Three-Phase Ic Measurement VSM A/RConn2 -- VSC VSM A/LConn2
  Three-Phase Ic Measurement VSM A/RConn3 -- VSC VSM A/LConn3
  Filter inductor VSM A/RConn2 -- Three-Phase Ic Measurement VSM A/LConn2
  Filter inductor VSM A/RConn1 -- Three-Phase Ic Measurement VSM A/LConn1
  Three-Phase Ic Measurement VSC A/RConn3 -- VSC A/LConn3
  Filter inductor VSM A/RConn3 -- Three-Phase Ic Measurement VSM A/LConn3
  Three-Phase Ic Measurement VSC A/RConn1 -- VSC A/LConn1
  Three-Phase Ic Measurement VSC A/RConn2 -- VSC A/LConn2
  Three-Phase Ic Measurement VSM A/RConn1 -- VSC VSM A/LConn1
  Three-Phase V-I Measurement Hotel Load A/LConn2 -- Three-Phase V-I Measurement 12puls  A3/RConn2 -- Three-Phase V-I Measurement 12puls  A1/RConn2 -- Three-Phase V-I Measurement 12puls  A2/LConn2 -- Three-Phase V-I Measurement 12puls  A/LConn2
  Three-Phase Vf Measurement VSM A/LConn1 -- Filter inductor 1 VSM A/RConn1
  Three-Phase Vf Measurement VSM A/LConn3 -- Filter inductor 1 VSM A/RConn3
  Filter inductor 1 VSM A/RConn2 -- Three-Phase Vf Measurement VSM A/LConn2
  Filter inductor 1 VSC A/RConn1 -- Three-Phase Vf Measurement VSC A/LConn1
  Three-Phase Vf Measurement VSC A/LConn2 -- Filter inductor 1 VSC A/RConn2
  Filter inductor 1 VSC A/RConn3 -- Three-Phase Vf Measurement VSC A/LConn3
  Three-Phase Bus Breaker SM A1/LConn3 -- Three-Phase Bus Breaker SM A/LConn3 -- Shunt resistor SM A/LConn3 -- Synchronous Machine A pu Fundamental/RConn3
  Shunt resistor SM A/LConn2 -- Three-Phase Bus Breaker SM A/LConn2 -- Three-Phase Bus Breaker SM A1/LConn2 -- Synchronous Machine A pu Fundamental/RConn2
  Three-Phase Bus Breaker SM A1/LConn1 -- Three-Phase Bus Breaker SM A/LConn1 -- Shunt resistor SM A/LConn1 -- Synchronous Machine A pu Fundamental/RConn1
  Shunt resistor SM A/RConn3 -- Shunt resistor SM A/RConn2 -- Shunt resistor SM A/RConn1
  Three-Phase Parallel RLC Snubber Load A/LConn1 -- Three-Phase Bus Breaker SM A1/RConn1
  Three-Phase Parallel RLC Snubber Load A/LConn2 -- Three-Phase Bus Breaker SM A1/RConn2
  Three-Phase Parallel RLC Snubber Load A/LConn3 -- Three-Phase Bus Breaker SM A1/RConn3
  Three-Phase V-I Measurement 12puls  A/RConn1 -- Three-Phase Transformer (Three Windings) 12puls A/LConn1
  Three-Phase V-I Measurement 12puls  A/RConn2 -- Three-Phase Transformer (Three Windings) 12puls A/LConn2
  Three-Phase V-I Measurement 12puls  A/RConn3 -- Three-Phase Transformer (Three Windings) 12puls A/LConn3
  Filter inductor VSC A/RConn1 -- Three-Phase Ic Measurement VSC A/LConn1
  Filter inductor VSC A/RConn2 -- Three-Phase Ic Measurement VSC A/LConn2
  Filter inductor VSC A/RConn3 -- Three-Phase Ic Measurement VSC A/LConn3
  Three-Phase Parallel RLC Load Hotel Load A/LConn1 -- Three-Phase V-I Measurement Hotel Load A/RConn1
  Three-Phase Parallel RLC Load Hotel Load A/LConn2 -- Three-Phase V-I Measurement Hotel Load A/RConn2
  Three-Phase Parallel RLC Load Hotel Load A/LConn3 -- Three-Phase V-I Measurement Hotel Load A/RConn3
  Three-Phase V-I Measurement 12puls  A1/LConn3 -- Filter inductor 1 VSM A/LConn3
  Three-Phase V-I Measurement 12puls  A1/LConn2 -- Filter inductor 1 VSM A/LConn2
  Three-Phase V-I Measurement 12puls  A1/LConn1 -- Filter inductor 1 VSM A/LConn1
  Three-Phase V-I Measurement 12puls  A2/RConn2 -- Filter inductor 1 VSC A/LConn2
  Three-Phase V-I Measurement 12puls  A2/RConn1 -- Filter inductor 1 VSC A/LConn1
  Three-Phase V-I Measurement 12puls  A2/RConn3 -- Filter inductor 1 VSC A/LConn3
  Three-Phase V-I Measurement Hotel Load A/LConn3 -- Three-Phase V-I Measurement 12puls  A3/RConn3 -- Three-Phase V-I Measurement 12puls  A/LConn3 -- Three-Phase V-I Measurement 12puls  A2/LConn3 -- Three-Phase V-I Measurement 12puls  A1/RConn3
  Three-Phase V-I Measurement Hotel Load A/LConn1 -- Three-Phase V-I Measurement 12puls  A3/RConn1 -- Three-Phase V-I Measurement 12puls  A1/RConn1 -- Three-Phase V-I Measurement 12puls  A2/LConn1 -- Three-Phase V-I Measurement 12puls  A/LConn1
  Three-Phase V-I Measurement 12puls  A3/LConn1 -- Three-Phase Bus Breaker SM A/RConn1
  Three-Phase V-I Measurement 12puls  A3/LConn2 -- Three-Phase Bus Breaker SM A/RConn2
  Three-Phase V-I Measurement 12puls  A3/LConn3 -- Three-Phase Bus Breaker SM A/RConn3

== system Simulation_model_islanded/Automatic Voltage Regulator SM A ==
  v_hat* : Inport
  v_hat_o : Inport  Port=2
  q* : Inport  Port=3
  qo : Inport  Port=4
  Gain15 : Gain  Gain=K_iv_SM
  Gain2 : Gain  Gain=Kq_SM
  Gain8 : Gain  Gain=K_pv_SM
  Integrator : Integrator  UpperSaturationLimit=10  LowerSaturationLimit=-10
  Sum1 : Sum  Inputs=-++
  Sum2 : Sum  Inputs=|+-
  Sum9 : Sum  Inputs=|++
  Transfer Fcn (with initial outputs) : simulink_extras/Additional Linear/Transfer Fcn (with initial outputs)  N=[omega_qf_SM]  D="[1  omega_qf_SM]"  Y0=0  U0=0
  v_hat_e : Outport
  wires:
  Integrator/1 -> Sum9/2
  Sum1/1 -> Gain15/1, Gain8/1
  Gain15/1 -> Integrator/1
  Gain8/1 -> Sum9/1
  q*/1 -> Sum2/1
  qo/1 -> Transfer Fcn (with initial outputs)/1
  Transfer Fcn (with initial outputs)/1 -> Sum2/2
  Sum2/1 -> Gain2/1
  v_hat*/1 -> Sum1/2
  Gain2/1 -> Sum1/3
  v_hat_o/1 -> Sum1/1
  Sum9/1 -> v_hat_e/1

== system Simulation_model_islanded/Diesel Generator Governor Model SM A ==
  p*_sm : Inport
  omega_sm* : Inport  Port=2
  omega_sm : Inport  Port=3
  Sum1 : Sum  Inputs=++|
  Sum2 : Sum  Inputs=|+-
  Transfer Fcn (with initial outputs)2 : simulink_extras/Additional Linear/Transfer Fcn (with initial outputs)  N=[1]  D=[T_gt_SM 1]  Y0=0  U0=0
  "k_omega, sm" : Gain  Gain=K_omega_SM
  tau_dg : Outport
  wires:
  omega_sm*/1 -> Sum2/1
  omega_sm/1 -> Sum2/2
  Sum2/1 -> "k_omega, sm"/1
  "k_omega, sm"/1 -> Sum1/2
  p*_sm/1 -> Sum1/1
  Sum1/1 -> Transfer Fcn (with initial outputs)2/1
  Transfer Fcn (with initial outputs)2/1 -> tau_dg/1

== system Simulation_model_islanded/P to I VSC A ==
  p_load : Inport
  v_dc : Inport  Port=2
  Divide : Product  Inputs=*/
  Transfer Fcn (with initial outputs) : simulink_extras/Additional Linear/Transfer Fcn (with initial outputs)  N=[5]  D="[1  5]"  Y0=1  U0=1
  i_dc : Outport
  wires:
  Divide/1 -> i_dc/1
  v_dc/1 -> Transfer Fcn (with initial outputs)/1
  p_load/1 -> Divide/1
  Transfer Fcn (with initial outputs)/1 -> Divide/2

== system Simulation_model_islanded/P to I 12puls A ==
  p* : Inport
  v_dc : Inport  Port=2
  Divide : Product  Inputs=*/
  Saturation : Saturate  UpperLimit=1.5  LowerLimit=0.5
  Transfer Fcn (with initial outputs) : simulink_extras/Additional Linear/Transfer Fcn (with initial outputs)  N=[20]  D="[1  20]"  Y0=1  U0=1
  i_dc : Outport
  wires:
  Divide/1 -> i_dc/1
  v_dc/1 -> Saturation/1
  Saturation/1 -> Transfer Fcn (with initial outputs)/1
  p*/1 -> Divide/1
  Transfer Fcn (with initial outputs)/1 -> Divide/2

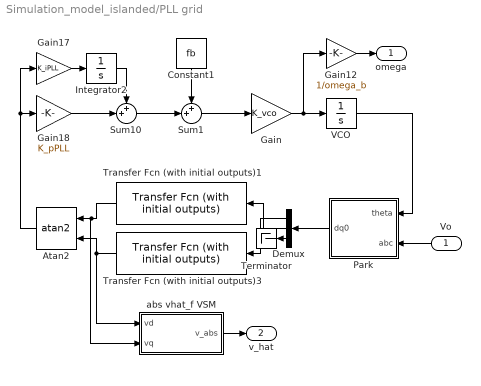
== system Simulation_model_islanded/PLL grid ==
  Vo : Inport
  Atan2 : Trigonometry  Operator=atan2  OutputSignalType=real
  Constant1 : Constant  Value=fb
  Demux : Demux  Outputs=3
  Gain : Gain  Gain=K_vco
  Gain12 : Gain  Gain=1/omega_b
  Gain17 : Gain  Gain=K_iPLL
  Gain18 : Gain  Gain=K_pPLL
  Integrator2 : Integrator
  Park : MATLAB Function  TreatAsAtomicUnit=on
  Sum1 : Sum  Inputs=++|
  Sum10 : Sum  Inputs=++|
  Terminator : Terminator
  Transfer Fcn (with initial outputs)1 : simulink_extras/Additional Linear/Transfer Fcn (with initial outputs)  N=[1]  D=[T_fPLL, 1]  Y0=0  U0=0
  Transfer Fcn (with initial outputs)3 : simulink_extras/Additional Linear/Transfer Fcn (with initial outputs)  N=[1]  D=[T_fPLL, 1]  Y0=1  U0=1
  VCO : Integrator  WrapState=on  WrappedStateUpperValue=2*pi  WrappedStateLowerValue=0
  abs vhat_f VSM : MATLAB Function  TreatAsAtomicUnit=on
  omega : Outport
  v_hat : Outport  Port=2
  wires:
  Transfer Fcn (with initial outputs)1/1 -> Atan2/1, abs vhat_f VSM/2(vq)
  Transfer Fcn (with initial outputs)3/1 -> Atan2/2, abs vhat_f VSM/1(vd)
  VCO/1 -> Park/1(theta)
  Sum1/1 -> Gain/1
  Gain/1 -> Gain12/1, VCO/1
  Constant1/1 -> Sum1/1
  Park/1(dq0) -> Demux/1
  Sum10/1 -> Sum1/2
  Atan2/1 -> Gain18/1, Gain17/1
  Demux/1 -> Transfer Fcn (with initial outputs)3/1
  Demux/2 -> Transfer Fcn (with initial outputs)1/1
  Vo/1 -> Park/2(abc)
  Gain18/1 -> Sum10/2
  Integrator2/1 -> Sum10/1
  Gain17/1 -> Integrator2/1
  Gain12/1 -> omega/1
  Demux/3 -> Terminator/1
  abs vhat_f VSM/1(v_abs) -> v_hat/1

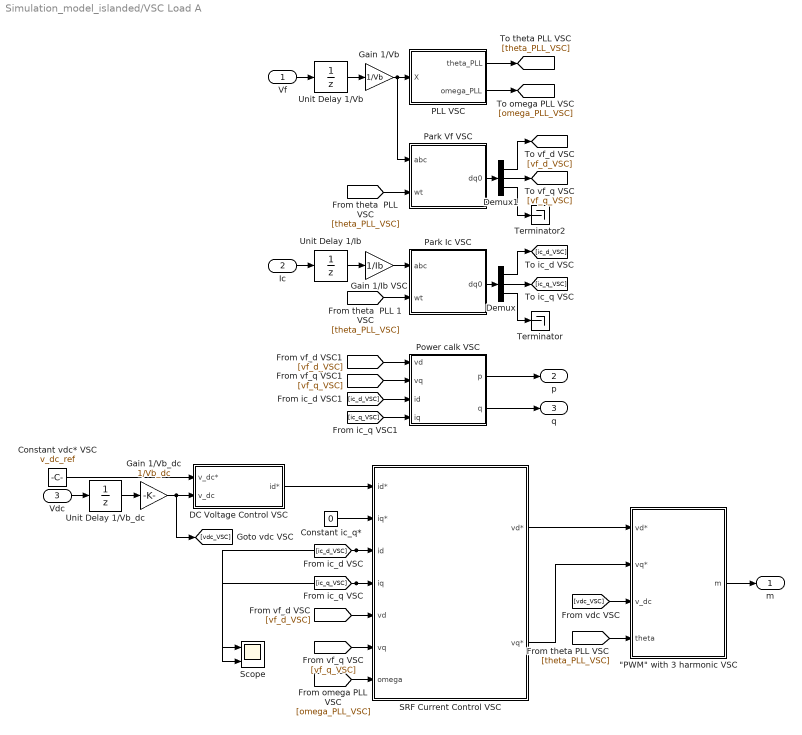
== system Simulation_model_islanded/VSC Load A ==
  Vf : Inport
  Ic : Inport  Port=2
  Vdc : Inport  Port=3
  "\"PWM\" with 3 harmonic VSC" : Subsystem
  Constant ic_q* : Constant  Value=0
  Constant vdc* VSC : Constant  Value=v_dc_ref
  DC Voltage Control VSC : Subsystem
  Demux : Demux  Outputs=3
  Demux1 : Demux  Outputs=3
  Gain 1/Ib VSC : Gain  Gain=1/Ib
  Gain 1/Vb : Gain  Gain=1/Vb
  Gain 1/Vb_dc : Gain  Gain=1/Vb_dc
  PLL VSC : Subsystem
  Park Ic VSC : MATLAB Function  TreatAsAtomicUnit=on
  Park Vf VSC : MATLAB Function  TreatAsAtomicUnit=on
  Power calk VSC : MATLAB Function  TreatAsAtomicUnit=on
  SRF Current Control VSC : Subsystem
  Scope : Scope  NumInputPorts=2
  Terminator : Terminator
  Terminator2 : Terminator
  Unit Delay 1/Ib : UnitDelay  SampleTime=-1  HasFrameUpgradeWarning=on
  Unit Delay 1/Vb : UnitDelay  SampleTime=-1  HasFrameUpgradeWarning=on
  "Unit Delay 1/Vb_dc " : UnitDelay  InitialCondition=Vb_dc  SampleTime=-1  HasFrameUpgradeWarning=on
  m : Outport
  p : Outport  Port=2
  q : Outport  Port=3
  wires:
  Constant vdc* VSC/1 -> DC Voltage Control VSC/1(v_dc*)
  [theta_PLL_VSC] -> Park Ic VSC/2(wt)
  Gain 1/Ib VSC/1 -> Park Ic VSC/1(abc)
  Vf/1 -> Unit Delay 1/Vb/1
  Gain 1/Vb_dc/1 -> [vdc_VSC], DC Voltage Control VSC/2(v_dc)
  [ic_d_VSC] -> Power calk VSC/3(id)
  Gain 1/Vb/1 -> Park Vf VSC/1(abc), PLL VSC/1(X)
  Demux1/2 -> [vf_q_VSC]
  [omega_PLL_VSC] -> SRF Current Control VSC/7(omega)
  Demux1/3 -> Terminator2/1
  [vf_d_VSC] -> Power calk VSC/1(vd)
  Park Ic VSC/1(dq0) -> Demux/1
  [ic_q_VSC] -> Power calk VSC/4(iq)
  PLL VSC/2(omega_PLL) -> [omega_PLL_VSC]
  PLL VSC/1(theta_PLL) -> [theta_PLL_VSC]
  SRF Current Control VSC/2(vq*) -> "\"PWM\" with 3 harmonic VSC"/2(vq*)
  [vf_q_VSC] -> SRF Current Control VSC/6(vq)
  Unit Delay 1/Ib/1 -> Gain 1/Ib VSC/1
  Park Vf VSC/1(dq0) -> Demux1/1
  [vf_q_VSC] -> Power calk VSC/2(vq)
  Demux1/1 -> [vf_d_VSC]
  [theta_PLL_VSC] -> "\"PWM\" with 3 harmonic VSC"/4(theta)
  Demux/1 -> [ic_d_VSC]
  Power calk VSC/1(p) -> p/1
  Unit Delay 1/Vb/1 -> Gain 1/Vb/1
  [theta_PLL_VSC] -> Park Vf VSC/2(wt)
  [ic_d_VSC] -> Scope/1, SRF Current Control VSC/3(id)
  [ic_q_VSC] -> SRF Current Control VSC/4(iq), Scope/2
  Demux/2 -> [ic_q_VSC]
  DC Voltage Control VSC/1(id*) -> SRF Current Control VSC/1(id*)
  SRF Current Control VSC/1(vd*) -> "\"PWM\" with 3 harmonic VSC"/1(vd*)
  Demux/3 -> Terminator/1
  [vdc_VSC] -> "\"PWM\" with 3 harmonic VSC"/3(v_dc)
  Constant ic_q*/1 -> SRF Current Control VSC/2(iq*)
  "Unit Delay 1/Vb_dc "/1 -> Gain 1/Vb_dc/1
  [vf_d_VSC] -> SRF Current Control VSC/5(vd)
  Ic/1 -> Unit Delay 1/Ib/1
  Vdc/1 -> "Unit Delay 1/Vb_dc "/1
  "\"PWM\" with 3 harmonic VSC"/1(m) -> m/1
  Power calk VSC/2(q) -> q/1

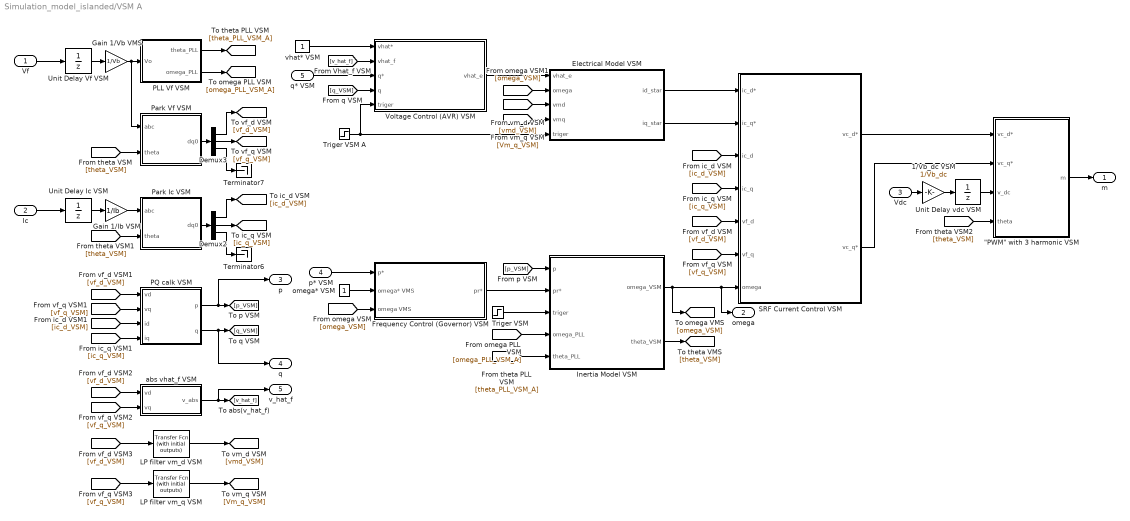
== system Simulation_model_islanded/VSM A ==
  Vf : Inport
  Ic : Inport  Port=2
  Vdc : Inport  Port=3
  p* VSM : Inport  Port=4
  q* VSM : Inport  Port=5
  "\"PWM\" with 3 harmonic VSM" : Subsystem
  1/Vb_dc VSM : Gain  Gain=1/Vb_dc
  Demux2 : Demux  Outputs=3
  Demux3 : Demux  Outputs=3
  Electrical Model VSM : MATLAB Function  TreatAsAtomicUnit=on
  Frequency Control (Governor) VSM : Subsystem
  Gain 1/Ib VSM : Gain  Gain=1/Ib
  Gain 1/Vb VMS : Gain  Gain=1/Vb
  Inertia Model VSM : Subsystem
  LP filter vm_d VSM : simulink_extras/Additional Linear/Transfer Fcn (with initial outputs)  N=[omega_vf]  D="[1  omega_vf]"  Y0=1  U0=1
  LP filter vm_q VSM : simulink_extras/Additional Linear/Transfer Fcn (with initial outputs)  N=[omega_vf]  D="[1  omega_vf]"  Y0=0  U0=0
  PLL Vf VSM : Subsystem
  PQ calk VSM : MATLAB Function  TreatAsAtomicUnit=on
  Park Ic VSM : MATLAB Function  TreatAsAtomicUnit=on
  Park Vf VSM : MATLAB Function  TreatAsAtomicUnit=on
  SRF Current Control VSM : Subsystem
  Terminator6 : Terminator
  Terminator7 : Terminator
  Triger VSM : Step  Time=0  Before=1  After=0  SampleTime=0
  Triger VSM A : Step  Time=0  Before=1  After=0  SampleTime=0
  Unit Delay Ic VSM : UnitDelay  SampleTime=-1  HasFrameUpgradeWarning=on
  Unit Delay Vf VSM : UnitDelay  SampleTime=-1  HasFrameUpgradeWarning=on
  Unit Delay vdc VSM : UnitDelay  InitialCondition=1  SampleTime=-1  HasFrameUpgradeWarning=on
  Voltage Control (AVR) VSM : Subsystem
  abs vhat_f VSM : MATLAB Function  TreatAsAtomicUnit=on
  omega* VSM : Constant
  vhat* VSM : Constant
  m : Outport
  omega : Outport  Port=2
  p : Outport  Port=3
  q : Outport  Port=4
  v_hat_f : Outport  Port=5
  wires:
  [theta_VSM] -> Park Vf VSM/2(theta)
  [theta_VSM] -> "\"PWM\" with 3 harmonic VSM"/4(theta)
  [vf_q_VSM] -> SRF Current Control VSM/6(vf_q)
  Demux3/1 -> [vf_d_VSM]
  [q_VSM] -> Voltage Control (AVR) VSM/4(q)
  [vf_d_VSM] -> PQ calk VSM/1(vd)
  SRF Current Control VSM/2(vc_q*) -> "\"PWM\" with 3 harmonic VSM"/2(vc_q*)
  Park Ic VSM/1(dq0) -> Demux2/1
  Vdc/1 -> 1/Vb_dc VSM/1
  Unit Delay vdc VSM/1 -> "\"PWM\" with 3 harmonic VSM"/3(v_dc)
  Vf/1 -> Unit Delay Vf VSM/1
  omega* VSM/1 -> Frequency Control (Governor) VSM/2(omega* VMS)
  [theta_VSM] -> Park Ic VSM/2(theta)
  Demux2/2 -> [ic_q_VSM]
  [omega_VSM] -> Frequency Control (Governor) VSM/3(omega VMS)
  LP filter vm_d VSM/1 -> [vmd_VSM]
  [ic_d_VSM] -> PQ calk VSM/3(id)
  [vf_d_VSM] -> abs vhat_f VSM/1(vd)
  LP filter vm_q VSM/1 -> [Vm_q_VSM]
  Demux3/3 -> Terminator7/1
  1/Vb_dc VSM/1 -> Unit Delay vdc VSM/1
  Inertia Model VSM/2(theta_VSM) -> [theta_VSM]
  [ic_q_VSM] -> PQ calk VSM/4(iq)
  [vf_q_VSM] -> LP filter vm_q VSM/1
  [vmd_VSM] -> Electrical Model VSM/3(vmd)
  [vf_q_VSM] -> abs vhat_f VSM/2(vq)
  "\"PWM\" with 3 harmonic VSM"/1(m) -> m/1
  [v_hat_f] -> Voltage Control (AVR) VSM/2(vhat_f)
  [ic_q_VSM] -> SRF Current Control VSM/4(ic_q)
  PLL Vf VSM/2(omega_PLL) -> [omega_PLL_VSM_A]
  p* VSM/1 -> Frequency Control (Governor) VSM/1(p*)
  [omega_PLL_VSM_A] -> Inertia Model VSM/4(omega_PLL)
  PLL Vf VSM/1(theta_PLL) -> [theta_PLL_VSM_A]
  Frequency Control (Governor) VSM/1(pr*) -> Inertia Model VSM/2(pr*)
  [theta_PLL_VSM_A] -> Inertia Model VSM/5(theta_PLL)
  Unit Delay Ic VSM/1 -> Gain 1/Ib VSM/1
  Triger VSM A/1 -> Voltage Control (AVR) VSM/5(triger), Electrical Model VSM/5(triger)
  q* VSM/1 -> Voltage Control (AVR) VSM/3(q*)
  Demux2/1 -> [ic_d_VSM]
  Voltage Control (AVR) VSM/1(vhat_e) -> Electrical Model VSM/1(vhat_e)
  [omega_VSM] -> Electrical Model VSM/2(omega)
  vhat* VSM/1 -> Voltage Control (AVR) VSM/1(vhat*)
  SRF Current Control VSM/1(vc_d*) -> "\"PWM\" with 3 harmonic VSM"/1(vc_d*)
  [vf_d_VSM] -> LP filter vm_d VSM/1
  Triger VSM/1 -> Inertia Model VSM/3(triger)
  Demux2/3 -> Terminator6/1
  [Vm_q_VSM] -> Electrical Model VSM/4(vmq)
  [vf_d_VSM] -> SRF Current Control VSM/5(vf_d)
  Inertia Model VSM/1(omega_VSM) -> [omega_VSM], SRF Current Control VSM/7(omega), omega/1
  [ic_d_VSM] -> SRF Current Control VSM/3(ic_d)
  Gain 1/Ib VSM/1 -> Park Ic VSM/1(abc)
  Demux3/2 -> [vf_q_VSM]
  [vf_q_VSM] -> PQ calk VSM/2(vq)
  Unit Delay Vf VSM/1 -> Gain 1/Vb VMS/1
  Park Vf VSM/1(dq0) -> Demux3/1
  abs vhat_f VSM/1(v_abs) -> v_hat_f/1, [v_hat_f]
  Ic/1 -> Unit Delay Ic VSM/1
  PQ calk VSM/1(p) -> p/1, [p_VSM]
  PQ calk VSM/2(q) -> q/1, [q_VSM]
  Gain 1/Vb VMS/1 -> Park Vf VSM/1(abc), PLL Vf VSM/1(Vo)
  Electrical Model VSM/1(id_star) -> SRF Current Control VSM/1(ic_d*)
  Electrical Model VSM/2(iq_star) -> SRF Current Control VSM/2(ic_q*)
  [p_VSM] -> Inertia Model VSM/1(p)

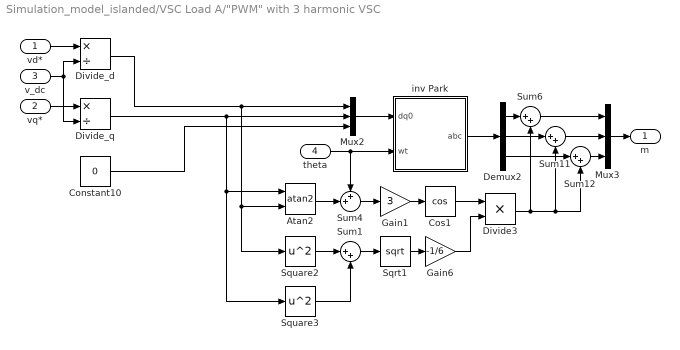
== system Simulation_model_islanded/VSC Load A/"PWM" with 3 harmonic VSC ==
  vd* : Inport
  vq* : Inport  Port=2
  v_dc : Inport  Port=3
  theta : Inport  Port=4
  Atan2 : Trigonometry  Operator=atan2
  Constant10 : Constant  Value=0
  Cos1 : Trigonometry  Operator=cos
  Demux2 : Demux  Outputs=3
  Divide3 : Product  Inputs=**
  Divide_d : Product  Inputs=*/
  Divide_q : Product  Inputs=*/
  Gain1 : Gain  Gain=3
  Gain6 : Gain  Gain=-1/6
  Mux2 : Mux  Inputs=3
  Mux3 : Mux  Inputs=3
  Sqrt1 : Sqrt  SaturateOnIntegerOverflow=on
  Square2 : Math  Operator=square  SaturateOnIntegerOverflow=on
  Square3 : Math  Operator=square  SaturateOnIntegerOverflow=on
  Sum{1,6,11..12} (4 alike) : Sum  Inputs=|++
  Sum4 : Sum  Inputs=++|
  inv Park : MATLAB Function  TreatAsAtomicUnit=on
  m : Outport
  wires:
  Constant10/1 -> Mux2/3
  Demux2/2 -> Sum11/1
  Sum4/1 -> Gain1/1
  Square2/1 -> Sum1/1
  Demux2/3 -> Sum12/1
  Divide3/1 -> Sum12/2, Sum11/2, Sum6/2
  Atan2/1 -> Sum4/2
  theta/1 -> Sum4/1, inv Park/2(wt)
  Gain6/1 -> Divide3/2
  Gain1/1 -> Cos1/1
  Sum12/1 -> Mux3/3
  Demux2/1 -> Sum6/1
  Sum6/1 -> Mux3/1
  Square3/1 -> Sum1/2
  Sum1/1 -> Sqrt1/1
  Cos1/1 -> Divide3/1
  Sum11/1 -> Mux3/2
  Sqrt1/1 -> Gain6/1
  Mux2/1 -> inv Park/1(dq0)
  vq*/1 -> Divide_q/1
  v_dc/1 -> Divide_d/2, Divide_q/2
  vd*/1 -> Divide_d/1
  Divide_d/1 -> Mux2/1, Atan2/2, Square2/1
  Divide_q/1 -> Square3/1, Atan2/1, Mux2/2
  Mux3/1 -> m/1
  inv Park/1(abc) -> Demux2/1

== system Simulation_model_islanded/VSC Load A/DC Voltage Control VSC ==
  v_dc* : Inport
  v_dc : Inport  Port=2
  Gain : Gain  Gain=-1
  Gain20 : Gain  Gain=K_idc
  Gain21 : Gain  Gain=K_pdc
  Integrator3 : Integrator
  Sum15 : Sum  Inputs=|++
  Sum16 : Sum  Inputs=|+-
  id* : Outport
  wires:
  Gain21/1 -> Sum15/1
  Sum16/1 -> Gain21/1, Gain20/1
  Integrator3/1 -> Sum15/2
  v_dc*/1 -> Sum16/1
  v_dc/1 -> Sum16/2
  Gain20/1 -> Integrator3/1
  Sum15/1 -> Gain/1
  Gain/1 -> id*/1

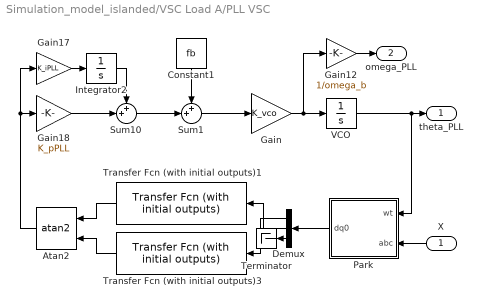
== system Simulation_model_islanded/VSC Load A/PLL VSC ==
  X : Inport
  Atan2 : Trigonometry  Operator=atan2  OutputSignalType=real
  Constant1 : Constant  Value=fb
  Demux : Demux  Outputs=3
  Gain : Gain  Gain=K_vco
  Gain12 : Gain  Gain=1/omega_b
  Gain17 : Gain  Gain=K_iPLL
  Gain18 : Gain  Gain=K_pPLL
  Integrator2 : Integrator
  Park : MATLAB Function  TreatAsAtomicUnit=on
  Sum1 : Sum  Inputs=++|
  Sum10 : Sum  Inputs=++|
  Terminator : Terminator
  Transfer Fcn (with initial outputs)1 : simulink_extras/Additional Linear/Transfer Fcn (with initial outputs)  N=[1]  D=[T_fPLL, 1]  Y0=0  U0=0
  Transfer Fcn (with initial outputs)3 : simulink_extras/Additional Linear/Transfer Fcn (with initial outputs)  N=[1]  D=[T_fPLL, 1]  Y0=1  U0=1
  VCO : Integrator  WrapState=on  WrappedStateUpperValue=2*pi  WrappedStateLowerValue=0
  theta_PLL : Outport
  omega_PLL : Outport  Port=2
  wires:
  Transfer Fcn (with initial outputs)1/1 -> Atan2/1
  Transfer Fcn (with initial outputs)3/1 -> Atan2/2
  VCO/1 -> theta_PLL/1, Park/1(wt)
  Sum1/1 -> Gain/1
  Gain/1 -> Gain12/1, VCO/1
  Constant1/1 -> Sum1/1
  Park/1(dq0) -> Demux/1
  Sum10/1 -> Sum1/2
  Atan2/1 -> Gain18/1, Gain17/1
  Demux/1 -> Transfer Fcn (with initial outputs)3/1
  Demux/2 -> Transfer Fcn (with initial outputs)1/1
  X/1 -> Park/2(abc)
  Gain18/1 -> Sum10/2
  Integrator2/1 -> Sum10/1
  Gain17/1 -> Integrator2/1
  Gain12/1 -> omega_PLL/1
  Demux/3 -> Terminator/1

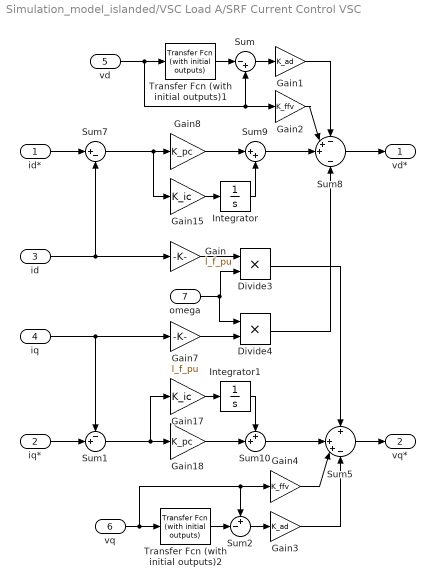
== system Simulation_model_islanded/VSC Load A/SRF Current Control VSC ==
  id* : Inport
  iq* : Inport  Port=2
  id : Inport  Port=3
  iq : Inport  Port=4
  vd : Inport  Port=5
  vq : Inport  Port=6
  omega : Inport  Port=7
  Divide3 : Product  Inputs=**
  Divide4 : Product  Inputs=**
  Gain : Gain  Gain=l_f_pu
  Gain1 : Gain  Gain=K_ad
  Gain15 : Gain  Gain=K_ic
  Gain17 : Gain  Gain=K_ic
  Gain18 : Gain  Gain=K_pc
  Gain2 : Gain  Gain=K_ffv
  Gain3 : Gain  Gain=K_ad
  Gain4 : Gain  Gain=K_ffv
  Gain7 : Gain  Gain=l_f_pu
  Gain8 : Gain  Gain=K_pc
  Integrator : Integrator  InitialCondition=1
  Integrator1 : Integrator
  Sum : Sum  Inputs=|-+
  Sum1 : Sum  Inputs=-+|
  Sum10 : Sum  Inputs=++|
  Sum2 : Sum  Inputs=+-|
  Sum5 : Sum  Inputs=+|++-
  Sum7 : Sum  Inputs=|+-
  Sum8 : Sum  Inputs=-++|-
  Sum9 : Sum  Inputs=|++
  Transfer Fcn (with initial outputs)1 : simulink_extras/Additional Linear/Transfer Fcn (with initial outputs)  N=[omega_ad]  D="[1  omega_ad]"  Y0=1  U0=1
  Transfer Fcn (with initial outputs)2 : simulink_extras/Additional Linear/Transfer Fcn (with initial outputs)  N=[omega_ad]  D="[1  omega_ad]"  Y0=0  U0=0
  vd* : Outport
  vq* : Outport  Port=2
  wires:
  iq*/1 -> Sum1/2
  Sum7/1 -> Gain15/1, Gain8/1
  Gain15/1 -> Integrator/1
  Sum1/1 -> Gain18/1, Gain17/1
  Divide3/1 -> Sum5/1
  Divide4/1 -> Sum8/4
  Gain7/1 -> Divide4/2
  Gain/1 -> Divide3/1
  Gain17/1 -> Integrator1/1
  Sum9/1 -> Sum8/3
  Integrator1/1 -> Sum10/1
  omega/1 -> Divide4/1, Divide3/2
  Gain18/1 -> Sum10/2
  Sum8/1 -> vd*/1
  Sum10/1 -> Sum5/2
  Gain8/1 -> Sum9/1
  iq/1 -> Gain7/1, Sum1/1
  Integrator/1 -> Sum9/2
  id/1 -> Gain/1, Sum7/2
  id*/1 -> Sum7/1
  Sum5/1 -> vq*/1
  Transfer Fcn (with initial outputs)1/1 -> Sum/1
  Sum/1 -> Gain1/1
  vd/1 -> Transfer Fcn (with initial outputs)1/1, Sum/2, Gain2/1
  Sum2/1 -> Gain3/1
  vq/1 -> Sum2/1, Gain4/1, Transfer Fcn (with initial outputs)2/1
  Transfer Fcn (with initial outputs)2/1 -> Sum2/2
  Gain4/1 -> Sum5/3
  Gain3/1 -> Sum5/4
  Gain2/1 -> Sum8/2
  Gain1/1 -> Sum8/1
